simulink model "p1_2"  (R2019b)
settings: Solver=VariableStepAuto  StartTime=0.0  StopTime=80.0  RelTol=1e-3
libraries: simulink x1
settings Model: Creator=ushio  LastModifiedBy=ushio

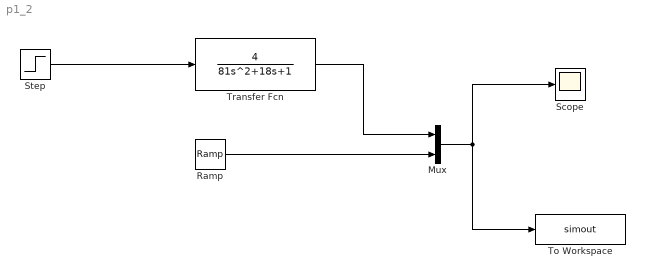
== system p1_2 ==
  Mux : Mux  Inputs=2
  Ramp : simulink/Sources/Ramp  slope=0.1635  start=2.535  InitialOutput=0
  Scope : Scope
  Step : Step  Time=0  SampleTime=0
  To Workspace : ToWorkspace  VariableName=simout  SaveFormat=Timeseries  SampleTime=-1
  Transfer Fcn : TransferFcn  Numerator=4  Denominator=[81 18 1]
  wires:
  Transfer Fcn/1 -> Mux/1
  Mux/1 -> To Workspace/1, Scope/1
  Step/1 -> Transfer Fcn/1
  Ramp/1 -> Mux/2
